simulink model "Realistic_scheme_2019_3"  (R2019b)
settings: Solver=VariableStepAuto  StartTime=0.0  StopTime=20  RelTol=1e-3
values from neighbouring files (symbols this model uses):
  A = [[0 0 1 0] ... (first row only)    [ClosedLoop.m]    (also in Inverted_pendulum.m; Realistic_model.m)
  B = [0 ... (first row only)    [ClosedLoop.m]    (also in Inverted_pendulum.m; Realistic_model.m)
  C = eye(n)    [ClosedLoop.m]    (also in Inverted_pendulum.m = [4.41/0.456, 0, 0, 0; Realistic_model.m = zeros(n,n); C(1,1) = 1; C(2,2) = 1)
  Con_from_V = [0.456/4.41, 0; 0, (pi/4)/6.328]    [Realistic_model.m]
  Con_to_V = [4.41/0.456, 0, 0, 0; 0, 6.328/(pi/4), 0, 0]    [Realistic_model.m]
  D = zeros(n,1)    [ClosedLoop.m]    (also in Inverted_pendulum.m = [0;0]; Realistic_model.m)
  Ts = 1/200    (= 0.005)    [Realistic_model.m]
  V_max_in = 5    [Realistic_model.m]
  V_max_out = 10    [Realistic_model.m]
  wc = 2*2*pi    (= 12.5663706144)    [Realistic_model.m]
undefined symbols (not defined in the file or in its folder): K
libraries: simulink x3
settings Model: Creator=elina  LastModifiedBy=gebruiker

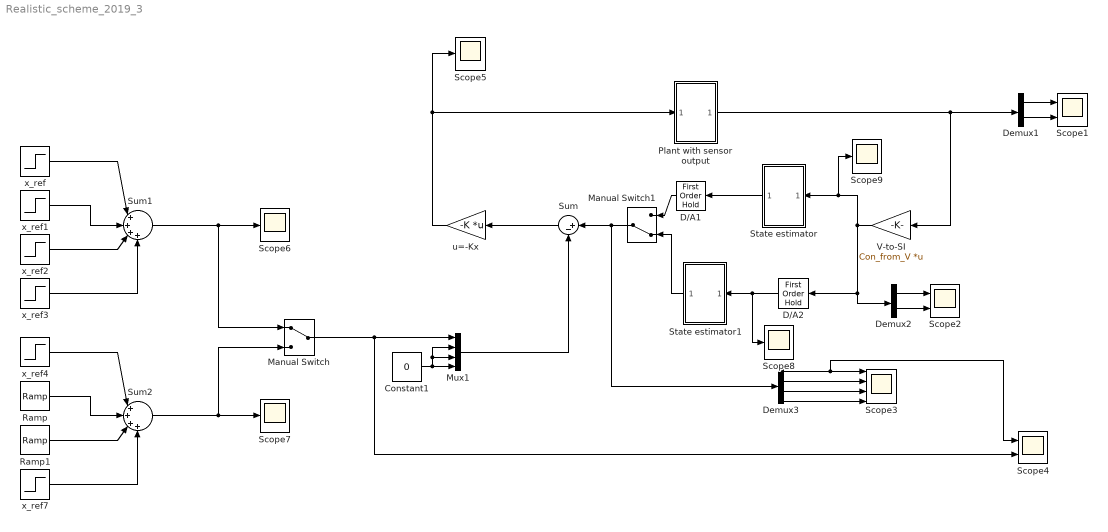
== system Realistic_scheme_2019_3 ==
  Constant1 : Constant  Value=0
  D/A1 : FirstOrderHold  OutputAlgorithm=Fast (Minimize Error)  ErrorTolerance=inf
  D/A2 : FirstOrderHold  OutputAlgorithm=Fast (Minimize Error)  ErrorTolerance=inf
  Demux1 : Demux  Outputs=2
  Demux2 : Demux  Outputs=2
  Demux3 : Demux
  Manual Switch : ManualSwitch
  Manual Switch1 : ManualSwitch  CurrentSetting=0
  Mux1 : Mux
  Plant with sensor output : Subsystem
  Ramp : simulink/Sources/Ramp  slope=1  start=15  InitialOutput=0
  Ramp1 : simulink/Sources/Ramp  slope=-1  start=17  InitialOutput=0
  Scope1 : Scope  NumInputPorts=2
  Scope2 : Scope  NumInputPorts=2
  Scope3 : Scope  NumInputPorts=4
  Scope4 : Scope  NumInputPorts=2
  Scope{5..9} (5 alike) : Scope
  State estimator : Subsystem
  State estimator1 : Subsystem
  Sum : Sum  Inputs=|+-
  Sum1 : Sum  Inputs=|++++
  Sum2 : Sum  Inputs=|++++
  V-to-SI : Gain  Gain=Con_from_V  Multiplication=Matrix(K*u)
  u=-Kx : Gain  Gain=-K  Multiplication=Matrix(K*u)
  x_ref : Step  Time=5  After=-1  SampleTime=0
  x_ref1 : Step  Time=9  After=1.25  SampleTime=0
  x_ref2 : Step  Time=8  After=0.25*0  SampleTime=0
  x_ref3 : Step  Time=15  After=0.35*0  SampleTime=0
  x_ref4 : Step  Time=11  After=-1  SampleTime=0
  x_ref7 : Step  Time=15  After=0.35*0  SampleTime=0
  wires:
  Constant1/1 -> Mux1/2, Mux1/3, Mux1/4
  Sum/1 -> u=-Kx/1
  V-to-SI/1 -> D/A2/1, Demux2/1, Scope9/1, State estimator/1(In1)
  Plant with sensor output/1(Out1) -> V-to-SI/1, Demux1/1
  Mux1/1 -> Sum/2
  Demux1/1 -> Scope1/1
  Demux1/2 -> Scope1/2
  Demux2/1 -> Scope2/1
  Demux2/2 -> Scope2/2
  u=-Kx/1 -> Scope5/1, Plant with sensor output/1(In1)
  State estimator/1(Out1) -> D/A1/1
  Demux3/1 -> Scope4/1, Scope3/1
  Demux3/2 -> Scope3/2
  Demux3/3 -> Scope3/3
  Demux3/4 -> Scope3/4
  x_ref3/1 -> Sum1/4
  x_ref2/1 -> Sum1/3
  x_ref1/1 -> Sum1/2
  x_ref/1 -> Sum1/1
  x_ref7/1 -> Sum2/4
  Ramp/1 -> Sum2/2
  x_ref4/1 -> Sum2/1
  Manual Switch/1 -> Scope4/2, Mux1/1
  Ramp1/1 -> Sum2/3
  Sum1/1 -> Scope6/1, Manual Switch/1
  Sum2/1 -> Scope7/1, Manual Switch/2
  D/A2/1 -> Scope8/1, State estimator1/1(In1)
  D/A1/1 -> Manual Switch1/1
  State estimator1/1(Out1) -> Manual Switch1/2
  Manual Switch1/1 -> Demux3/1, Sum/1

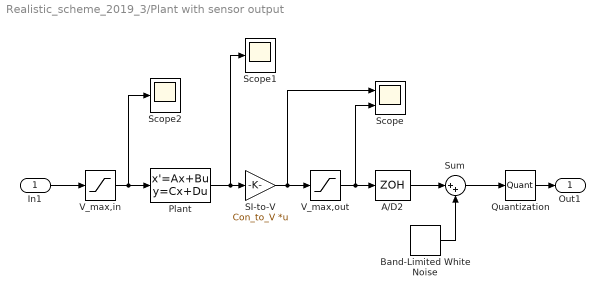
== system Realistic_scheme_2019_3/Plant with sensor output ==
  In1 : Inport
  A/D2 : ZeroOrderHold  SampleTime=Ts
  Band-Limited White Noise : simulink/Sources/Band-Limited White Noise  Cov=10e-7  Ts=Ts  seed=[23341]
  Plant : StateSpace  A=A  B=B  C=C  D=D  InitialCondition=[-0.5, 25*pi/180, 0, 0]
  Quantization : Quantizer  QuantizationInterval=quant_step
  SI-to-V : Gain  Gain=Con_to_V  Multiplication=Matrix(K*u)
  Scope : Scope  NumInputPorts=2
  Scope1 : Scope
  Scope2 : Scope
  Sum : Sum  Inputs=|++
  V_max,in : Saturate  UpperLimit=V_max_in  LowerLimit=-V_max_in
  V_max,out : Saturate  UpperLimit=V_max_out  LowerLimit=-V_max_out
  Out1 : Outport
  wires:
  Plant/1 -> Scope1/1, SI-to-V/1
  V_max,out/1 -> Scope/2, A/D2/1
  SI-to-V/1 -> Scope/1, V_max,out/1
  Quantization/1 -> Out1/1
  A/D2/1 -> Sum/1
  Sum/1 -> Quantization/1
  Band-Limited White Noise/1 -> Sum/2
  In1/1 -> V_max,in/1
  V_max,in/1 -> Scope2/1, Plant/1

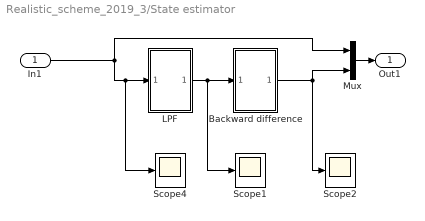
== system Realistic_scheme_2019_3/State estimator ==
  In1 : Inport
  Backward difference : Subsystem
  LPF : Subsystem
  Mux : Mux  Inputs=2
  Scope1 : Scope
  Scope2 : Scope
  Scope4 : Scope
  Out1 : Outport
  wires:
  LPF/1(Out1) -> Scope1/1, Backward difference/1(In1)
  Backward difference/1(Out1) -> Scope2/1, Mux/2
  Mux/1 -> Out1/1
  In1/1 -> Mux/1, Scope4/1, LPF/1(In1)

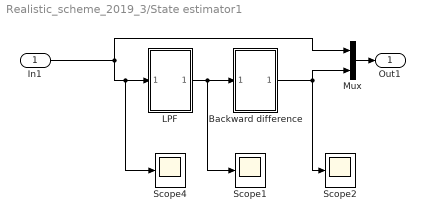
== system Realistic_scheme_2019_3/State estimator1 ==
  In1 : Inport
  Backward difference : Subsystem
  LPF : Subsystem
  Mux : Mux  Inputs=2
  Scope1 : Scope
  Scope2 : Scope
  Scope4 : Scope
  Out1 : Outport
  wires:
  LPF/1(Out1) -> Scope1/1, Backward difference/1(In1)
  Backward difference/1(Out1) -> Scope2/1, Mux/2
  Mux/1 -> Out1/1
  In1/1 -> Mux/1, Scope4/1, LPF/1(In1)

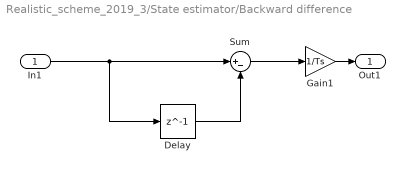
== system Realistic_scheme_2019_3/State estimator/Backward difference ==
  In1 : Inport
  Delay : Delay  DelayLength=1  InitialCondition=0
  Gain1 : Gain  Gain=1/Ts
  Sum : Sum  Inputs=|+-
  Out1 : Outport
  wires:
  Delay/1 -> Sum/2
  Gain1/1 -> Out1/1
  In1/1 -> Delay/1, Sum/1
  Sum/1 -> Gain1/1

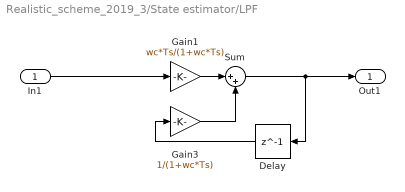
== system Realistic_scheme_2019_3/State estimator/LPF ==
  In1 : Inport
  Delay : Delay  DelayLength=1
  Gain1 : Gain  Gain=wc*Ts/(1+wc*Ts)
  Gain3 : Gain  Gain=1/(1+wc*Ts)
  Sum : Sum  Inputs=|++
  Out1 : Outport
  wires:
  Gain3/1 -> Sum/2
  Sum/1 -> Out1/1, Delay/1
  Delay/1 -> Gain3/1
  In1/1 -> Gain1/1
  Gain1/1 -> Sum/1

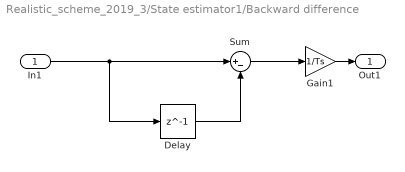
== system Realistic_scheme_2019_3/State estimator1/Backward difference ==
  In1 : Inport
  Delay : Delay  DelayLength=1  InitialCondition=0
  Gain1 : Gain  Gain=1/Ts
  Sum : Sum  Inputs=|+-
  Out1 : Outport
  wires:
  Delay/1 -> Sum/2
  Gain1/1 -> Out1/1
  In1/1 -> Delay/1, Sum/1
  Sum/1 -> Gain1/1

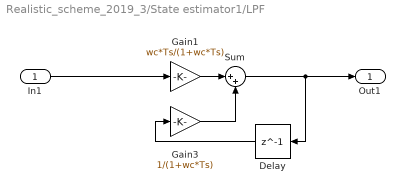
== system Realistic_scheme_2019_3/State estimator1/LPF ==
  In1 : Inport
  Delay : Delay  DelayLength=1
  Gain1 : Gain  Gain=wc*Ts/(1+wc*Ts)
  Gain3 : Gain  Gain=1/(1+wc*Ts)
  Sum : Sum  Inputs=|++
  Out1 : Outport
  wires:
  Gain3/1 -> Sum/2
  Sum/1 -> Out1/1, Delay/1
  Delay/1 -> Gain3/1
  In1/1 -> Gain1/1
  Gain1/1 -> Sum/1
